simulink model "dfir_df"  (R2023b)
settings: Solver=VariableStepAuto  StartTime=0.0  StopTime=10.0  RelTol=1e-3
undefined symbols (not defined in the file): a1, a2, b0, b1, b2
settings Model: Creator=eechris  LastModifiedBy=eechris

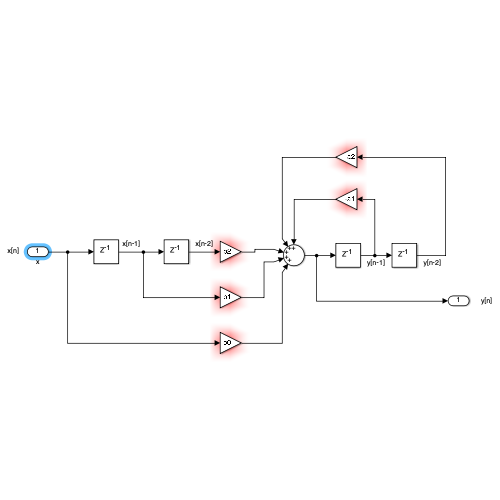
[thumbnail: Simulink's stored preview of the top-level diagram]
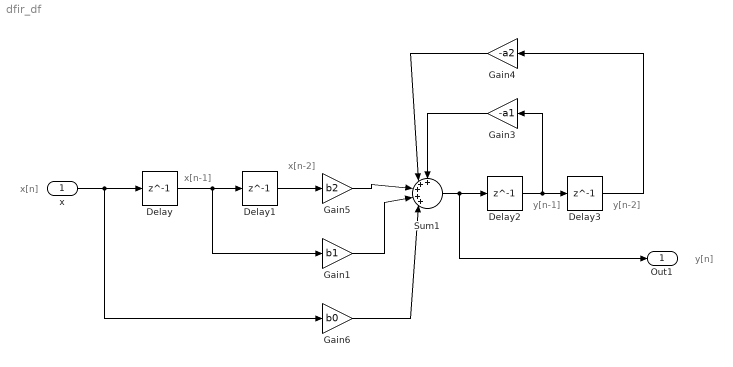
== system dfir_df ==
  note: x[n]
  note: y[n]
  note: x[n-1]
  note: x[n-2]
  note: y[n-1]
  note: y[n-2]
  x : Inport
  Delay{,1..3} (4 alike) : Delay  DelayLength=1  InitialCondition=0
  Gain1 : Gain  Gain=b1
  Gain3 : Gain  Gain=-a1
  Gain4 : Gain  Gain=-a2
  Gain5 : Gain  Gain=b2
  Gain6 : Gain  Gain=b0
  Sum1 : Sum  Inputs=+++++|
  Out1 : Outport
  wires:
  Delay/1 -> Gain1/1, Delay1/1
  x/1 -> Gain6/1, Delay/1
  Delay1/1 -> Gain5/1
  Gain5/1 -> Sum1/3
  Gain6/1 -> Sum1/5
  Gain1/1 -> Sum1/4
  Sum1/1 -> Out1/1, Delay2/1
  Delay2/1 -> Gain3/1, Delay3/1
  Delay3/1 -> Gain4/1
  Gain3/1 -> Sum1/1
  Gain4/1 -> Sum1/2
